simulink model "Week2_prob3"  (R2020b)
settings: Solver=VariableStepAuto  StartTime=0.0  StopTime=120.0  RelTol=1e-3
values from neighbouring files (symbols this model uses):
  b = 50.0    [Data_dictionary_prob3.sldd]
  m = 1000.0    [Data_dictionary_prob3.sldd]
undefined symbols (not defined in the file or in its folder): Ki, Kp, Ts
settings Model: Creator=Lakshmi  LastModifiedBy=Lakshmi

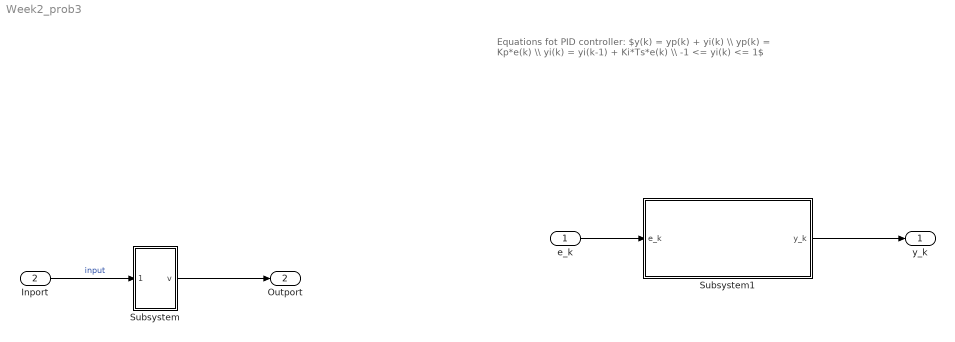
== system Week2_prob3 ==
  note: Equations fot PID controller:
      | $y(k) = yp(k) + yi(k) \\ yp(k) = Kp*e(k) \\ yi(k) = yi(k-1) + Ki*Ts*e(k) \\ -1 <= yi(k) <= 1$
  e_k : Inport
  Inport : Inport  Port=2
  Subsystem : Subsystem
  Subsystem1 : Subsystem
  y_k : Outport
  Outport : Outport  Port=2
  wires:
  Inport/1 -> Subsystem/1(input)  "input"
  Subsystem/1(v) -> Outport/1
  e_k/1 -> Subsystem1/1(e_k)
  Subsystem1/1(y_k) -> y_k/1

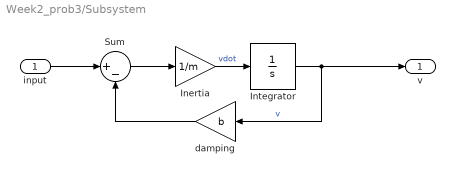
== system Week2_prob3/Subsystem ==
  input : Inport
  Inertia : Gain  Gain=1/m
  Integrator : Integrator
  Sum : Sum  Inputs=|+-
  damping : Gain  Gain=b
  v : Outport
  wires:
  Sum/1 -> Inertia/1
  input/1 -> Sum/1
  Integrator/1 -> v/1, damping/1  "v"
  damping/1 -> Sum/2
  Inertia/1 -> Integrator/1  "vdot"

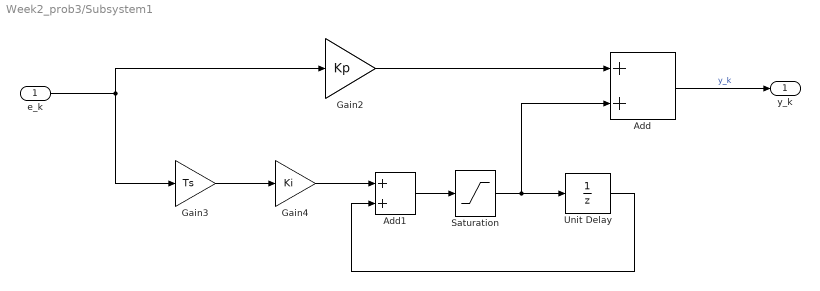
== system Week2_prob3/Subsystem1 ==
  e_k : Inport
  Add : Sum
  Add1 : Sum
  Gain2 : Gain  Gain=Kp
  Gain3 : Gain  Gain=Ts
  Gain4 : Gain  Gain=Ki
  Saturation : Saturate
  Unit Delay : UnitDelay  SampleTime=-1  HasFrameUpgradeWarning=on
  y_k : Outport
  wires:
  Gain2/1 -> Add/1
  Gain4/1 -> Add1/1
  Add1/1 -> Saturation/1
  e_k/1 -> Gain2/1, Gain3/1
  Gain3/1 -> Gain4/1
  Unit Delay/1 -> Add1/2
  Saturation/1 -> Unit Delay/1, Add/2
  Add/1 -> y_k/1  "y_k"
